simulink model "mass_fk_example_sim"  (R2025a)
settings: Solver=FixedStepAuto  StartTime=0.0  StopTime=10.0  FixedStep=1e-3  RelTol=1e-3
undefined symbols (not defined in the file): c, k
libraries: fl_lib x5, nesl_utility x4, simulink x2, sdl_lib x1
settings Model: Creator=amoralesma  LastModifiedBy=amoralesma

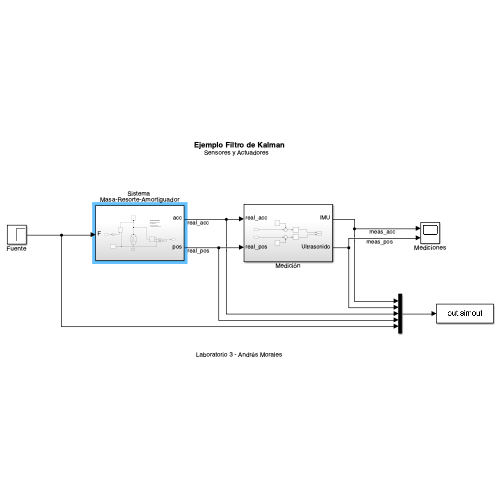
[thumbnail: Simulink's stored preview of the top-level diagram]
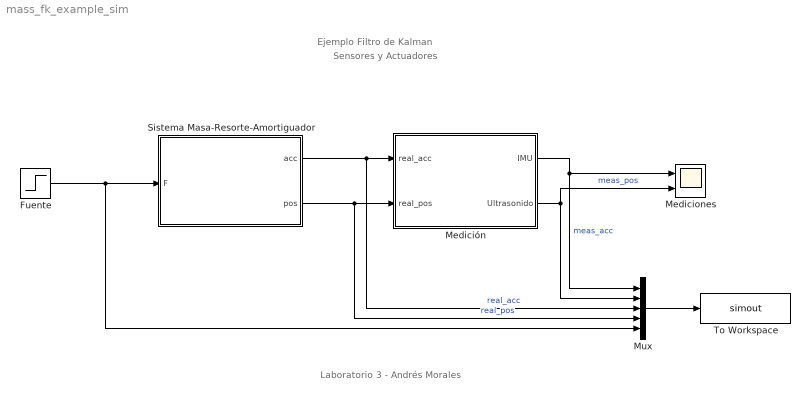
== system mass_fk_example_sim ==
  note: Ejemplo Filtro de Kalman
  note: Sensores y Actuadores
  note: Laboratorio 3 - Andrés Morales
  Fuente : Step  Time=0  SampleTime=0
  Mediciones : Scope  NumInputPorts=2
      settings: ActiveDisplayYMinimum=-0.87350817662507507  ActiveDisplayYMaximum=1.1808640506203083
  Medición : Subsystem
  Mux : Mux  Inputs=5
  Sistema Masa-Resorte-Amortiguador : Subsystem
  To Workspace : ToWorkspace  VariableName=simout  SaveFormat=Timeseries  SampleTime=-1
  wires:
  Fuente/1 -> Mux/5, Sistema Masa-Resorte-Amortiguador/1(F)
  Mux/1 -> To Workspace/1
  Medición/1(IMU) -> Mediciones/1, Mux/1  "meas_acc"
  Medición/2(Ultrasonido) -> Mux/2, Mediciones/2  "meas_pos"
  Sistema Masa-Resorte-Amortiguador/1(acc) -> Mux/3, Medición/1(real_acc)  "real_acc"
  Sistema Masa-Resorte-Amortiguador/2(pos) -> Mux/4, Medición/2(real_pos)  "real_pos"

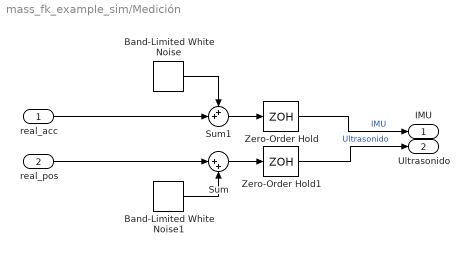
== system mass_fk_example_sim/Medición ==
  real_acc : Inport
  real_pos : Inport  Port=2
  Band-Limited White Noise : simulink/Sources/Band-Limited White Noise  Cov=[0.00001]  Ts=0.001  seed=[23341]
  Band-Limited White Noise1 : simulink/Sources/Band-Limited White Noise  Cov=[0.00001]  Ts=0.023  seed=[23341]
  Sum : Sum  Inputs=|++
  Sum1 : Sum  Inputs=++|
  Zero-Order Hold : ZeroOrderHold  SampleTime=-1
  Zero-Order Hold1 : ZeroOrderHold  SampleTime=-1
  IMU : Outport
  Ultrasonido : Outport  Port=2
  wires:
  real_acc/1 -> Sum1/2
  Zero-Order Hold1/1 -> Ultrasonido/1  "Ultrasonido"
  Zero-Order Hold/1 -> IMU/1  "IMU"
  Band-Limited White Noise/1 -> Sum1/1
  Band-Limited White Noise1/1 -> Sum/2
  real_pos/1 -> Sum/1
  Sum1/1 -> Zero-Order Hold/1
  Sum/1 -> Zero-Order Hold1/1

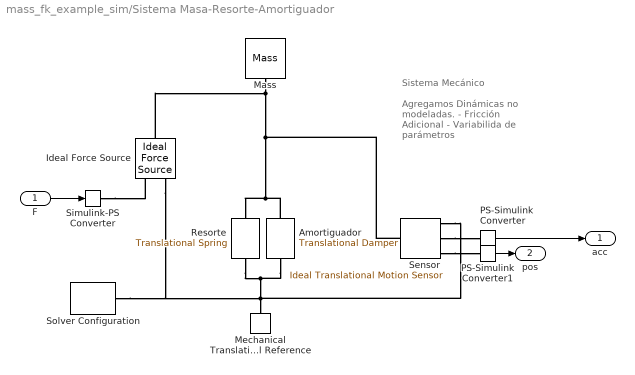
== system mass_fk_example_sim/Sistema Masa-Resorte-Amortiguador ==
  note: Agregamos Dinámicas
      | no modeladas.
      |
      | - Fricción Adicional
      | - Variabilida de parámetros
  note: Sistema Mecánico
  F : Inport
  Amortiguador : sdl_lib/Couplings & Drives/Springs & Dampers/Translational Damper  D=c * 0.9 N*s/m  thermal_port=simscape.enum.thermaleffects.omit  thermal_mass=50 kJ/K  temperature_specify=off  temperature_priority=High  temperature=300 K  temperature_nominal_specify=off  temperature_nominal_value=1  temperature_nominal_unit=K
  Ideal Force Source : fl_lib/Mechanical/Mechanical Sources/Ideal Force Source
  Mass : fl_lib/Mechanical/Translational Elements/Mass  mass=1 * 1.05 kg  num_ports=foundation.enum.numPorts2.one  v_specify=off  v_priority=High  v=0 m/s  v_nominal_specify=off  v_nominal_value=1  v_nominal_unit=m/s  f_specify=off  f_priority=None  f=0 N  f_nominal_specify=off  f_nominal_value=1  f_nominal_unit=N
  Mechanical Translational Reference : fl_lib/Mechanical/Translational Elements/Mechanical Translational Reference
  PS-Simulink Converter : nesl_utility/PS-Simulink Converter  PhysicalDomain=network_engine_domain  SubClassName=ps_output  LeftPortType=input  RightPortType=output  PseudoPeriodic=off  Frequencies=[]  VectorFormat=inherit  Unit=inherit  AffineConversion=off
  PS-Simulink Converter1 : nesl_utility/PS-Simulink Converter  PhysicalDomain=network_engine_domain  SubClassName=ps_output  LeftPortType=input  RightPortType=output  PseudoPeriodic=off  Frequencies=[]  VectorFormat=inherit  Unit=inherit  AffineConversion=off
  Resorte : fl_lib/Mechanical/Translational Elements/Translational Spring  spr_rate=k * 1.05 N/m  v_specify=off  v_priority=None  v=0 m/s  v_nominal_specify=off  v_nominal_value=1  v_nominal_unit=m/s  f_specify=off  f_priority=None  f=0 N  f_nominal_specify=off  f_nominal_value=1  f_nominal_unit=N  x_specify=off  x_priority=High  x=0 m  x_nominal_specify=off  x_nominal_value=0  x_nominal_unit=m
  Sensor : fl_lib/Mechanical/Mechanical Sensors/Ideal Translational Motion Sensor  reference=foundation.enum.MeasurementReference.difference  acceleration_port=true  velocity_port=false  position_port=true  offset=0 m
      settings: InternalSimscapePortConfiguration="{\"Bottom\":[],\"Left\":[{\"id\":\"R\",\"label\":\"R\",\"type\":\"foundation.mechanical.translational.translational\"}],\"Right\":[{\"id\":\"C\",\"label\":\"C\",\"type\":\"foundation.mechanical.translational.translational\"},{\"id\":\"A\",\"label\":\"A\",\"type\":\"output\"},{\"id\":\"P\",\"label\":\"P\",\"type\":\"output\"}],\"Top\":[]}"
  Simulink-PS Converter : nesl_utility/Simulink-PS Converter  PhysicalDomain=network_engine_domain  SubClassName=ps_input  LeftPortType=input  RightPortType=output  PseudoPeriodic=off  Frequencies=[]  NoiseDistribution=none  NoiseParameters=[]  Unit=1  AffineConversion=off  FilteringAndDerivatives=provide  SimscapeFilterOrder=1  InputFilterTimeConstant=0.001  UdotUserProvided=0
  Solver Configuration : nesl_utility/Solver Configuration  PhysicalDomain=network_engine_domain  SubClassName=solver  LeftPortType=input  RightPortType=generic  Tones=[]  Harmonics=[]  SimulateNoise=off  Profile=off  UseLocalSampling=off  EnableSwitchedLinearOptims=on  FrequencyDomain=off  UseCCode=off  RelTol=0.001  AbsTol=0.001  MinStep=1e-09  ToWorkspace=off  RevertToSquareIcSolve=off  NumHomotopyIterations=100  PhasorMode=off  PhasorModeNumHarmonics=1  ConsistencySolver=NEWTON_XTOL_AFTER_FTOL  IndexReductionMethod=DerivativeReplacement  DoDC=off  ResidualTolerance=1e-09  ConsistencyTolSource=GLOBAL  ConsistencyAbsTol=0.001  ConsistencyRelTol=0.001  ConsistencyTolFactor=0.001  UseLocalSolver=off  LocalSolverChoice=NE_BACKWARD_EULER_ADVANCER  ResolveIndetEquations=on  FunctionEvalNumThread=1  LocalSolverSampleTime=0.001  DoFixedCost=off  MaxNonlinIter=3  MaxModeIter=2  ComputeImpulses=off  ImpulseIterations=2  LinearAlgebra=auto  LinearAlgebraNumThread=0  EquationFormulation=NE_TIME_EF  DelaysMemoryBudget=1024  AutomaticFiltering=on  FilteringTimeConstant=0.001  PartitionStorageMethod=AS_NEEDED  PartitionMemoryBudget=1024  PartitionMethod=ROBUST  MultibodyUseLocalSolver=off  MultibodyLocalSolverChoice=ODE1  MultibodyLocalSolverSampleTime=0.001
  acc : Outport
  pos : Outport  Port=2
  wires:
  PS-Simulink Converter/1 -> acc/1
  PS-Simulink Converter1/1 -> pos/1
  F/1 -> Simulink-PS Converter/1
  connections:
  Resorte/LConn1 -- Amortiguador/RConn1 -- Sensor/RConn1 -- Ideal Force Source/RConn2 -- Solver Configuration/RConn1 -- Mechanical Translational Reference/LConn1
  Mass/LConn1 -- Ideal Force Source/LConn1 -- Sensor/LConn1 -- Amortiguador/LConn1 -- Resorte/RConn1
  Sensor/RConn3 -- PS-Simulink Converter1/LConn1
  Sensor/RConn2 -- PS-Simulink Converter/LConn1
  Simulink-PS Converter/RConn1 -- Ideal Force Source/RConn1
